simulink model "UAVIntegratedNavigationSystem"  (R2020b)
settings: Solver=FixedStepAuto  StartTime=0.0  StopTime=TFinal  FixedStep=IMUtime  RelTol=1e-3
values from neighbouring files (symbols this model uses):
  AIONtime = 1    [ModelSettings.m]
  BiasAccel = 9.81E-4    (= 0.000981)    [ModelSettings.m]
  BiasGyro = 2.424068405548E-4    (= 0.000242406840555)    [ModelSettings.m]
  CorrTimeOrientationGNSS = 1    [ModelSettings.m]
  CorrTimePositionGNSS = 1    [ModelSettings.m]
  CorrTimeVelocityGNSS = 1    [ModelSettings.m]
  delay = 1.5    [ModelSettings.m]
  e = 0.081819106    [ModelSettings.m]
  g0 = 9.780327    [ModelSettings.m]
  GNSStime = 0.2    [ModelSettings.m]
  H0 = 0.1    [ModelSettings.m]
  IMUtime = 0.01    [ModelSettings.m]
  indUAV = 2    [ModelSettings.m]
  LambdaInit = 0.6555    [ModelSettings.m]
  mass = 0.7    [ModelSettings.m]
  N = 100    [ModelSettings.m]
  PhiInit = 0.968    [ModelSettings.m]
  PitchDown = -PitchUp    (= -0.1)    [ModelSettings.m]
  PitchUp = 0.1    [ModelSettings.m]
  Ra = 6378.245    [ModelSettings.m]
  RollDown = -RollUp    (= -0.1)    [ModelSettings.m]
  RollUp = 0.1    [ModelSettings.m]
  SigmaAccel = 9.81E-4    (= 0.000981)    [ModelSettings.m]
  SigmaAION = 30    [ModelSettings.m]
  SigmaAltitudeGNSS = 3    [ModelSettings.m]
  SigmaGyro = 2.666475246102E-6    (= 2.6664752461e-06)    [ModelSettings.m]
  SigmaLaser = 5    [ModelSettings.m]
  SigmaOrientationGNSS = 0.00349    [ModelSettings.m]
  SigmaPositionGNSS = 1.5    [ModelSettings.m]
  SigmaVelocityGNSS = 0.03    [ModelSettings.m]
  SigmaVelocityUpGNSS = 0.03    [ModelSettings.m]
  U1down = 0    [ModelSettings.m]
  U1up = 4 * ForceCoeff * OmegaMax^2    (= 9.9858124)    [ModelSettings.m]
  U2down = -U2up    (= -2.4964531)    [ModelSettings.m]
  U2up = ForceCoeff * OmegaMax^2    (= 2.4964531)    [ModelSettings.m]
  U3down = -U3up    (= -2.4964531)    [ModelSettings.m]
  U3up = ForceCoeff * OmegaMax^2    (= 2.4964531)    [ModelSettings.m]
  U4down = -U4up    (= -0.2494604)    [ModelSettings.m]
  U4up = 2 * DragCoeff * OmegaMax^2    (= 0.2494604)    [ModelSettings.m]
  WEarth = 7.2921158553E-5    (= 7.2921158553e-05)    [ModelSettings.m]
undefined symbols (not defined in the file or in its folder): deg, Newton, rad, Raphson, s
libraries: simulink x11, sharedtransform x7, pid_lib x6, aerolibconvert2 x4, sharedutil x4
(part 5 of 5)

== matlab function UAVIntegratedNavigationSystem/Subsystem/Слабосвязанная схема комплексирования ИНС + ГНСС/MATLAB Function - FullLowCoastLinearKalman ==
  settings: updateMethod=DISCRETE
  data: Measure input; EstimateError output size=15; XError data_store_memory; PCovarianceError data_store_memory; I data_store_memory; H data_store_memory; RCovarianceMeasurement data_store_memory; timeGNSS data_store_memory; timeIMU data_store_memory; AltitudeSeaLevel data_store_memory; PhiEstimate data_store_memory; WEarth data_store_memory; QCovarianceSystem data_store_memory; Ell data_store_memory; StatusGNSS input; EstimateCovariance output size=15; C input
function [EstimateError, EstimateCovariance] = LowCoastKalman(Measure, StatusGNSS, C)
%% Входные данные:
% Measure - вектор измерений [9 x 1]
%           |    X_Geo_IMU - X_Geo_GNSS   |
%           |    Y_Geo_IMU - Y_Geo_GNSS   |
% Measure = |    Z_Geo_IMU - Z_Geo_GNSS   |
%           |  V_X_Geo_IMU - V_X_Geo_GNSS |
%           |  V_Y_Geo_IMU - V_Y_Geo_GNSS |
%           |  V_Z_Geo_IMU - V_Z_Geo_GNSS |
%           |     Roll_IMU - Roll_GNSS    |
%           |     Yaw_IMU  - Yaw_GNSS     |
%           |    Pitch_IMU - Pitch_GNSS   | 
% StatusGNSS - статус работы приемника ГНСС
% C - матрица перевода из связ. С.К. --> геогр. С.К.
%% Глобальные переменные
% Вектор состояния системы [15 x 1]
global XError;
% Апостериорная матрица ковариации [15 x 15]
global PCovarianceError;
% Единичная матрица [15 x 15]
global I;
% Матрица наблюдаемости [9 x 15]
global H;
% Матрица ковариации шумов измерений [9 x 9]
global RCovarianceMeasurement;
% Матрица ковариации шумов системы [6 x 6]
global QCovarianceSystem;
% Время дискретизации ИНС
global timeIMU; 
% Высота над уровнем моря, м
global AltitudeSeaLevel;
% Оценка широты, рад
global PhiEstimate;
% Угловая скорость вращения Земли, рад / сек
global WEarth;
% Параметры эллипсоида
global Ell;
%% Обновление широты
R1 = Ell(1) * (1 - Ell(2)^2) / ((1 - Ell(2)^2 * sin(PhiEstimate)^2)^1.5) + AltitudeSeaLevel * 10^3;
R2 = Ell(1)  / ((1 - Ell(2)^2 * sin(PhiEstimate)^2)^0.5) + AltitudeSeaLevel * 10^3;
PhiEstimate = PhiEstimate + XError(1) * timeIMU / R1;
%% Системные матрицы
% Матрица системы [15 x 15]
      %dNorth' %dHeight' %dEast'                           %dV_North'                                      %dV_Height'                                        %dV_East'                                     %dRoll'                 %dYaw'                        %dPitch'            %dAccX'         %dAccY'           %dAccZ'              %dGyroX'        %dGyroY'            %dGyroZ'    
A = [    0,       0,       0,                                  1,                                             0,                                                 0,                                           0,                      0,                            0,                   0,              0,               0,                  0,               0,                  0;...       %|     dNorth     |
         0,       0,       0,                                  0,                                             1,                                                 0,                                           0,                      0,                            0,                   0,              0,               0,                  0,               0,                  0;...       %|     dHeight    | 
         0,       0,       0,                                  0,                                             0,                                                 1,                                           0,                      0,                            0,                   0,              0,               0,                  0,               0,                  0;...       %|     dEast      |
         0,       0,       0,                          - XError(5) / R1,                                -XError(4)/ R1,      - XError(6) * tan(PhiEstimate) / R2 - 2 * WEarth * sin(PhiEstimate),             0,                      0,                            0,                 C(1,1),         C(1,2),          C(1,3),                0,              0,                  0;...       %|    dV_North    |
         0,       0,       0,                - XError(4) * tan(PhiEstimate)/ R2,                              0,                             XError(6) / R2 - 2 * WEarth * cos(PhiEstimate),                  0,                      0,                            0,                 C(2,1),         C(2,2),          C(2,3),                0,              0,                  0;...       %|    dV_Height   |
         0,       0,       0,    XError(6) * tan(PhiEstimate) / R2 + 2 * WEarth * sin(PhiEstimate), 2 * WEarth * cos(PhiEstimate),     XError(4) * tan(PhiEstimate)/ R2 - XError(5)/ R1,                      0,                      0,                            0,                 C(3,1),         C(3,2),          C(3,3),                0,              0,                  0;...       %|    dV_East     |
         0,       0,       0,                                   0,                                             0,                                                  0,                                         0,                      0,                            0,                    0,               0,               0,                C(1,1),         C(1,2),             C(1,3);...    %|     dRoll      |
         0,       0,       0,                                   0,                                             0,                                                  0,                                         0,                      0,                            0,                    0,               0,               0,                C(2,1),         C(2,2),             C(2,3);...    %|     dYaw       |
         0,       0,       0,                                   0,                                             0,                                                  0,                                         0,                      0,                            0,                    0,               0,               0,                C(3,1),         C(3,2),             C(3,3);...    %|     dPitch     |
         0,       0,       0,                                   0,                                             0,                                                  0,                                         0,                      0,                            0,                    0,               0,               0,                 0,               0,                  0;...       %|     dAccX      |
         0,       0,       0,                                   0,                                             0,                                                  0,                                         0,                      0,                            0,                    0,               0,               0,                 0,               0,                  0;...       %|     dAccY      |
         0,       0,       0,                                   0,                                             0,                                                  0,                                         0,                      0,                            0,                    0,               0,               0,                 0,               0,                  0;...       %|     dAccZ      | 
         0,       0,       0,                                   0,                                             0,                                                  0,                                         0,                      0,                            0,                    0,               0,               0,                 0,               0,                  0;...       %|     dGyroX     |
         0,       0,       0,                                   0,                                             0,                                                  0,                                         0,                      0,                            0,                    0,               0,               0,                 0,               0,                  0;...       %|     dGyroY     |   
         0,       0,       0,                                   0,                                             0,                                                  0,                                         0,                      0,                            0,                    0,               0,               0,                 0,               0,                  0];         %|     dGyroZ     | 
% Фундаментальная матрица системы [15 x 15]
F = I + timeIMU * A;
% Матрица шумов системы [15 x 6]
        %Noise_dAcc_X    %Noise_dAcc_Y    %Noise_dAcc_Z  %Noise_dGyro_X       %Noise_dGyro_Y       %Noise_dGyro_Z
G = timeIMU *[     0,               0,               0,               0,                   0,                  0;...            %|     dNorth    |
              0,               0,               0,               0,                   0,                  0;...            %|     dHeight   |
              0,               0,               0,               0,                   0,                  0;...            %|     dEast     |
            C(1,1),          C(1,2),           C(1,3),           0,                   0,                  0;...            %|    dV_North   |
            C(2,1),          C(2,2),           C(2,3),           0,                   0,                  0;...            %|    dV_Height  |
            C(3,1),          C(3,2),           C(3,3),           0,                   0,                  0;...            %|    dV_East    |
              0,               0,               0,              C(1,1),              C(1,2),             C(1,3);...        %|     dRoll     |
              0,               0,               0,              C(2,1),              C(2,2),             C(2,3);...        %|     dYaw      |
              0,               0,               0,              C(3,1),              C(3,2),             C(3,3);...        %|     dPitch    |
              0,               0,               0,               0,                    0,                 0;...            %|     dAccX     |
              0,               0,               0,               0,                    0,                 0;...            %|     dAccY     |
              0,               0,               0,               0,                    0,                 0;...            %|     dAccZ     |
              0,               0,               0,               0,                    0,                 0;...            %|     dGyroX    |
              0,               0,               0,               0,                    0,                 0;...            %|     dGyroY    |
              0,               0,               0,               0,                    0,                 0];              %|     dGyroZ    |
%% Прогноз - коррекция с помошью ГНСС
if ((StatusGNSS == 1))
% Коррекция вектора состояния
S = (H * PCovarianceError * H' + RCovarianceMeasurement)^(-1);
K = PCovarianceError * H' * S;
XError = XError + K * (Measure(:) - H * XError); 
PCovarianceError = (I - K * H) * PCovarianceError; 
else
% Прогноз вектора состояния
XError = F * XError;
PCovarianceError = F * PCovarianceError * F' + G * QCovarianceSystem * G';
end
%% Выходные переменные: Оценки вектора состояния и апостериорной ковариационной матрицы 
EstimateError = XError;
EstimateCovariance = [3 * sqrt(PCovarianceError(1,1)); 3 * sqrt(PCovarianceError(2,2));...
                      3 * sqrt(PCovarianceError(3,3)); 3 * sqrt(PCovarianceError(4,4));...
                      3 * sqrt(PCovarianceError(5,5)); 3 * sqrt(PCovarianceError(6,6));...
                      3 * sqrt(PCovarianceError(7,7)); 3 * sqrt(PCovarianceError(8,8));...
                      3 * sqrt(PCovarianceError(9,9)); 3 * sqrt(PCovarianceError(10,10));...
                      3 * sqrt(PCovarianceError(11,11)); 3 * sqrt(PCovarianceError(12,12));...
                      3 * sqrt(PCovarianceError(13,13)); 3 * sqrt(PCovarianceError(14,14));...
                      3 * sqrt(PCovarianceError(15,15))];

== matlab function UAVIntegratedNavigationSystem/Блок создания траектории движения БЛА/Параметры для моделирования квадрокоптера/MATLAB Function ==
  data: t input; Alt output; TAltitude input
function Alt = QuadroAltitude(t, TAltitude)
if ((t>=0) && (t<3))
     Alt = 5;
 elseif ((t>=3) && (t<15))  
     Alt = 10;
 elseif ((t>=15) && (t<25))  
     Alt = 20;
 elseif ((t>=25) && (t<30))  
     Alt = 30;     
 elseif ((t>=30) && (t<35))  
     Alt = 40;  
 elseif ((t>=35) && (t<50))  
     Alt = 50; 
 elseif ((t>=50) && (t<65))  
     Alt = 60; 
 elseif ((t>=65) && (t<75))  
     Alt = 70; 
 elseif ((t>=75) && (t<85))  
     Alt = 80; 
 elseif ((t>=85) && (t<TAltitude))  
     Alt = 100;
else
     Alt = 100;
end

== matlab function UAVIntegratedNavigationSystem/Subsystem/Слабосвязанная схема комплексирования ИНС + АИОН/MATLAB Function - LowCoastLinearKalmanPositionVelocity ==
  settings: updateMethod=DISCRETE
  data: Measure input; EstimateError output size=15; XError data_store_memory; PCovarianceError data_store_memory; I data_store_memory; H data_store_memory; RCovarianceMeasurement data_store_memory; timeIMU data_store_memory; AltitudeSeaLevel data_store_memory; PhiEstimate data_store_memory; WEarth data_store_memory; QCovarianceSystem data_store_memory; Ell data_store_memory; StatusAION input; EstimateCovariance output size=15; C input
function [EstimateError, EstimateCovariance] = LowCoastKalman(Measure, StatusAION, C)
%% Входные данные:
% Measure - вектор измерений [9 x 1]
%           |    X_Geo_IMU - X_Geo_AION   |
% Measure = |    Y_Geo_IMU - Y_Geo_AION   |
%           |    Z_Geo_IMU - Z_Geo_AION   |
% StatusAION - статус работы АИОН
% C - матрица перевода из связ. С.К. --> геогр. С.К.
%% Глобальные переменные
% Вектор состояния системы [15 x 1]
global XError;
% Апостериорная матрица ковариации [15 x 15]
global PCovarianceError;
% Единичная матрица [15 x 15]
global I;
% Матрица наблюдаемости [9 x 15]
global H;
% Матрица ковариации шумов измерений [9 x 9]
global RCovarianceMeasurement;
% Матрица ковариации шумов системы [6 x 6]
global QCovarianceSystem;
% Время дискретизации ИНС
global timeIMU; 
% Высота над уровнем моря, м
global AltitudeSeaLevel;
% Оценка широты, рад
global PhiEstimate;
% Угловая скорость вращения Земли, рад / сек
global WEarth;
% Параметры эллипсоида
global Ell;
%% Обновление широты
R1 = Ell(1) * (1 - Ell(2)^2) / ((1 - Ell(2)^2 * sin(PhiEstimate)^2)^1.5) + AltitudeSeaLevel * 10^3;
R2 = Ell(1)  / ((1 - Ell(2)^2 * sin(PhiEstimate)^2)^0.5) + AltitudeSeaLevel * 10^3;
PhiEstimate = PhiEstimate + XError(1) * timeIMU / R1;
%% Системные матрицы
% Матрица системы [15 x 15]
      %dNorth' %dHeight' %dEast'                           %dV_North'                                      %dV_Height'                                        %dV_East'                                     %dRoll'                 %dYaw'                        %dPitch'            %dAccX'         %dAccY'           %dAccZ'              %dGyroX'        %dGyroY'            %dGyroZ'    
A = [    0,       0,       0,                                  1,                                             0,                                                 0,                                           0,                      0,                            0,                   0,              0,               0,                  0,               0,                  0;...       %|     dNorth     |
         0,       0,       0,                                  0,                                             1,                                                 0,                                           0,                      0,                            0,                   0,              0,               0,                  0,               0,                  0;...       %|     dHeight    | 
         0,       0,       0,                                  0,                                             0,                                                 1,                                           0,                      0,                            0,                   0,              0,               0,                  0,               0,                  0;...       %|     dEast      |
         0,       0,       0,                          - XError(5) / R1,                                -XError(4)/ R1,      - XError(6) * tan(PhiEstimate) / R2 - 2 * WEarth * sin(PhiEstimate),             0,                      0,                            0,                 C(1,1),         C(1,2),          C(1,3),                0,              0,                  0;...       %|    dV_North    |
         0,       0,       0,                - XError(4) * tan(PhiEstimate)/ R2,                              0,                             XError(6) / R2 - 2 * WEarth * cos(PhiEstimate),                  0,                      0,                            0,                 C(2,1),         C(2,2),          C(2,3),                0,              0,                  0;...       %|    dV_Height   |
         0,       0,       0,    XError(6) * tan(PhiEstimate) / R2 + 2 * WEarth * sin(PhiEstimate), 2 * WEarth * cos(PhiEstimate),     XError(4) * tan(PhiEstimate)/ R2 - XError(5)/ R1,                      0,                      0,                            0,                 C(3,1),         C(3,2),          C(3,3),                0,              0,                  0;...       %|    dV_East     |
         0,       0,       0,                                   0,                                             0,                                                  0,                                         0,                      0,                            0,                    0,               0,               0,                C(1,1),         C(1,2),             C(1,3);...    %|     dRoll      |
         0,       0,       0,                                   0,                                             0,                                                  0,                                         0,                      0,                            0,                    0,               0,               0,                C(2,1),         C(2,2),             C(2,3);...    %|     dYaw       |
         0,       0,       0,                                   0,                                             0,                                                  0,                                         0,                      0,                            0,                    0,               0,               0,                C(3,1),         C(3,2),             C(3,3);...    %|     dPitch     |
         0,       0,       0,                                   0,                                             0,                                                  0,                                         0,                      0,                            0,                    0,               0,               0,                 0,               0,                  0;...       %|     dAccX      |
         0,       0,       0,                                   0,                                             0,                                                  0,                                         0,                      0,                            0,                    0,               0,               0,                 0,               0,                  0;...       %|     dAccY      |
         0,       0,       0,                                   0,                                             0,                                                  0,                                         0,                      0,                            0,                    0,               0,               0,                 0,               0,                  0;...       %|     dAccZ      | 
         0,       0,       0,                                   0,                                             0,                                                  0,                                         0,                      0,                            0,                    0,               0,               0,                 0,               0,                  0;...       %|     dGyroX     |
         0,       0,       0,                                   0,                                             0,                                                  0,                                         0,                      0,                            0,                    0,               0,               0,                 0,               0,                  0;...       %|     dGyroY     |   
         0,       0,       0,                                   0,                                             0,                                                  0,                                         0,                      0,                            0,                    0,               0,               0,                 0,               0,                  0];         %|     dGyroZ     | 
% Фундаментальная матрица системы [15 x 15]
F = I + timeIMU * A;
% Матрица шумов системы [15 x 6]
        %Noise_dAcc_X    %Noise_dAcc_Y    %Noise_dAcc_Z  %Noise_dGyro_X       %Noise_dGyro_Y       %Noise_dGyro_Z
G = timeIMU *[     0,               0,               0,               0,                   0,                  0;...            %|     dNorth    |
              0,               0,               0,               0,                   0,                  0;...            %|     dHeight   |
              0,               0,               0,               0,                   0,                  0;...            %|     dEast     |
            C(1,1),          C(1,2),           C(1,3),           0,                   0,                  0;...            %|    dV_North   |
            C(2,1),          C(2,2),           C(2,3),           0,                   0,                  0;...            %|    dV_Height  |
            C(3,1),          C(3,2),           C(3,3),           0,                   0,                  0;...            %|    dV_East    |
              0,               0,               0,              C(1,1),              C(1,2),             C(1,3);...        %|     dRoll     |
              0,               0,               0,              C(2,1),              C(2,2),             C(2,3);...        %|     dYaw      |
              0,               0,               0,              C(3,1),              C(3,2),             C(3,3);...        %|     dPitch    |
              0,               0,               0,               0,                    0,                 0;...            %|     dAccX     |
              0,               0,               0,               0,                    0,                 0;...            %|     dAccY     |
              0,               0,               0,               0,                    0,                 0;...            %|     dAccZ     |
              0,               0,               0,               0,                    0,                 0;...            %|     dGyroX    |
              0,               0,               0,               0,                    0,                 0;...            %|     dGyroY    |
              0,               0,               0,               0,                    0,                 0];              %|     dGyroZ    |
%% Прогноз - коррекция с помошью АИОН
if ((StatusAION == 1))
% Коррекция вектора состояния
S = (H * PCovarianceError * H' + RCovarianceMeasurement)^(-1);
K = PCovarianceError * H' * S;
XError = XError + K * (Measure(:) - H * XError); 
PCovarianceError = (I - K * H) * PCovarianceError; 
else
% Прогноз вектора состояния
XError = F * XError;
PCovarianceError = F * PCovarianceError * F' + G * QCovarianceSystem * G';
end
%% Выходные переменные: Оценки вектора состояния и апостериорной ковариационной матрицы 
EstimateError = XError;
EstimateCovariance = [3 * sqrt(PCovarianceError(1,1)); 3 * sqrt(PCovarianceError(2,2));...
                      3 * sqrt(PCovarianceError(3,3)); 3 * sqrt(PCovarianceError(4,4));...
                      3 * sqrt(PCovarianceError(5,5)); 3 * sqrt(PCovarianceError(6,6));...
                      3 * sqrt(PCovarianceError(7,7)); 3 * sqrt(PCovarianceError(8,8));...
                      3 * sqrt(PCovarianceError(9,9)); 3 * sqrt(PCovarianceError(10,10));...
                      3 * sqrt(PCovarianceError(11,11)); 3 * sqrt(PCovarianceError(12,12));...
                      3 * sqrt(PCovarianceError(13,13)); 3 * sqrt(PCovarianceError(14,14));...
                      3 * sqrt(PCovarianceError(15,15))];

== matlab function UAVIntegratedNavigationSystem/Блок создания траектории движения БЛА/Параметры для моделирования самолета типа 2/MATLAB Function2 ==
  data: t input; Alt output; TAltitude input
function Alt = WingFixedUAVAltitude(t, TAltitude)
if ((t>=0) && (t<3))
     Alt = 5;
 elseif ((t>=3) && (t<15))  
     Alt = 10;
 elseif ((t>=15) && (t<30))  
     Alt = 30;
 elseif ((t>=30) && (t<45))  
     Alt = 50;     
 elseif ((t>=45) && (t<60))  
     Alt = 70;  
 elseif ((t>=60) && (t<75))  
     Alt = 100; 
 elseif ((t>=75) && (t<90))  
     Alt = 130; 
 elseif ((t>=90) && (t<105))  
     Alt = 150; 
 elseif ((t>=105) && (t<120))  
     Alt = 170; 
 elseif ((t>=120) && (t<135))  
     Alt = 200;
elseif ((t>=135) && (t<150))
     Alt = 220;
elseif ((t>=150) && (t<165))
    Alt = 240;
elseif((t>=165) && (t<180))
    Alt = 260;
elseif ((t>=180) && (t<195))
    Alt = 280;
elseif ((t>195) && (t<TAltitude))
    Alt =300;
else
    Alt = 300;
end

== matlab function UAVIntegratedNavigationSystem/Блок создания траектории движения БЛА/Параметры для моделирования самолета типа 1/MATLAB Function2 ==
  data: t input; Alt output; TAltitude input
function Alt = WingFixedUAVAltitude(t, TAltitude)
if ((t>=0) && (t<3))
     Alt = 5;
 elseif ((t>=3) && (t<15))  
     Alt = 10;
 elseif ((t>=15) && (t<30))  
     Alt = 30;
 elseif ((t>=30) && (t<45))  
     Alt = 50;     
 elseif ((t>=45) && (t<60))  
     Alt = 70;  
 elseif ((t>=60) && (t<75))  
     Alt = 100; 
 elseif ((t>=75) && (t<90))  
     Alt = 130; 
 elseif ((t>=90) && (t<105))  
     Alt = 150; 
 elseif ((t>=105) && (t<120))  
     Alt = 170; 
 elseif ((t>=120) && (t<135))  
     Alt = 200;
elseif ((t>=135) && (t<150))
     Alt = 220;
elseif ((t>=150) && (t<165))
    Alt = 240;
elseif((t>=165) && (t<180))
    Alt = 260;
elseif ((t>=180) && (t<195))
    Alt = 280;
elseif ((t>195) && (t<TAltitude))
    Alt =300;
else
    Alt = 300;
end

== matlab function UAVIntegratedNavigationSystem/Блок модели динамики квадрокоптера + САУ/Полетный контроллер/Удержание положения/Обратная матрица  ==
  data: u input; y output
function y = fcn(u)
y = inv(u);

== matlab function UAVIntegratedNavigationSystem/Subsystem/MATLAB Function ==
  data: INSGNSS input; CorrectionVector output; INSAINS input; INS input; indKOI input
function CorrectionVector = fcn(INSGNSS, INSAINS, INS, indKOI)
if (indKOI == 1)
    CorrectionVector = INSGNSS;
elseif (indKOI == 2)
    CorrectionVector = INSAINS;
else
    CorrectionVector = INS;
end

== matlab function UAVIntegratedNavigationSystem/Subsystem1/Функционирование приемника ГНСС/MATLAB Function ==
  settings: updateMethod=DISCRETE
  data: GNSSStatus input; y output; sum data_store_memory
function y = fcn(GNSSStatus)
global sum;
if (GNSSStatus == -1)
    sum = sum + 1;
    y = sum;
else
    y = 0;
    sum = 0;
end

== matlab function UAVIntegratedNavigationSystem/Блок создания траектории движения БЛА/Выбор траектории движения БЛА/Eight Path ==
  data: X output; Z output; t input; NorthEight input; TAltitude input
function [X, Z]  = fcn(t, NorthEight, TAltitude)
X = NorthEight * cos((t - TAltitude) / 120);
Z = NorthEight * sin(2 * (t - TAltitude) / 120)/2;
end

== matlab function UAVIntegratedNavigationSystem/Блок создания траектории движения БЛА/Выбор траектории движения БЛА/Line Path ==
  data: X output; Z output; t input; TAltitude input
function [X, Z]  = fcn(t, TAltitude)
X = (t - TAltitude);
Z = (t - TAltitude);
end

== matlab function UAVIntegratedNavigationSystem/Блок создания траектории движения БЛА/Выбор траектории движения БЛА/Snake Path ==
  data: X output; Z output; t input; TAltitude input
function [X, Z]  = fcn(t, TAltitude)
X = 2000 * (1 - cos((t - TAltitude)/45))/2;
Z = ((t - TAltitude) - sin(t - TAltitude));
end

== matlab function UAVIntegratedNavigationSystem/Subsystem1/Функционирование АИОН/MATLAB Function ==
  settings: updateMethod=DISCRETE
  data: AIONStatus input; y output; sum data_store_memory
function y = fcn(AIONStatus)
global sum;
if (AIONStatus == -1)
    sum = sum + 1;
    y = sum;
else
    y = 0;
    sum = 0;
end
